simulink model "adaptive"  (R2018a)
settings: Solver=ode1  StartTime=0.0  StopTime=20  FixedStep=0.001  RelTol=1e-3
settings Model: Creator=mesih  LastModifiedBy=mesih

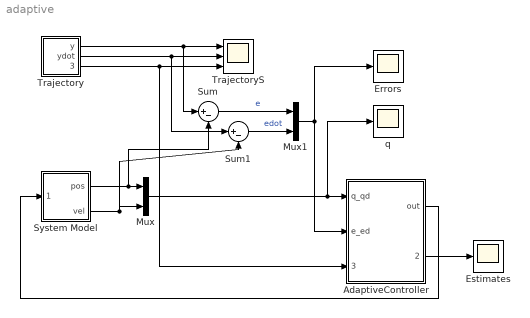
== system adaptive ==
  AdaptiveController : Subsystem
  Errors : Scope
  Estimates : Scope
  Mux : Mux  Inputs=2
  Mux1 : Mux  Inputs=2
  Sum : Sum  Inputs=|+-
  Sum1 : Sum  Inputs=|+-
  System Model : Subsystem
  Trajectory : Subsystem
  TrajectoryS : Scope  NumInputPorts=3
  q : Scope
  wires:
  Trajectory/1(y) -> Sum/1, TrajectoryS/1
  Trajectory/2(ydot) -> TrajectoryS/2, Sum1/1
  Trajectory/3(yddot) -> AdaptiveController/3(trajectory_dd), TrajectoryS/3
  System Model/1(pos) -> Sum/2, Mux/1
  System Model/2(vel) -> Mux/2, Sum1/2
  Sum/1 -> Mux1/1  "e"
  Sum1/1 -> Mux1/2  "edot"
  Mux1/1 -> AdaptiveController/2(e_ed), Errors/1
  AdaptiveController/1(out) -> System Model/1(input)
  Mux/1 -> q/1, AdaptiveController/1(q_qd)
  AdaptiveController/2("estimates ") -> Estimates/1

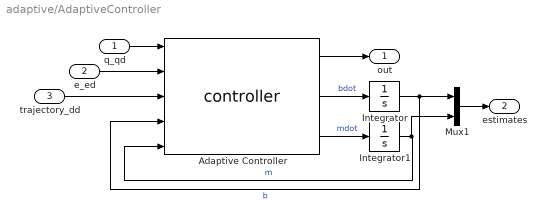
== system adaptive/AdaptiveController ==
  q_qd : Inport
  e_ed : Inport  Port=2
  trajectory_dd : Inport  Port=3
  Adaptive Controller : S-Function  FunctionName=controller  Parameters=1,10,5,3,0,0  SFunctionDeploymentMode=off  EnableBusSupport=off
  Integrator : Integrator
  Integrator1 : Integrator
  Mux1 : Mux  Inputs=2
  out : Outport
  "estimates " : Outport  Port=2
  wires:
  Adaptive Controller/1 -> out/1
  Integrator/1 -> Mux1/1, Adaptive Controller/4  "b"
  Integrator1/1 -> Mux1/2, Adaptive Controller/5  "m"
  Adaptive Controller/3 -> Integrator1/1  "mdot"
  q_qd/1 -> Adaptive Controller/1
  Adaptive Controller/2 -> Integrator/1  "bdot"
  trajectory_dd/1 -> Adaptive Controller/3
  e_ed/1 -> Adaptive Controller/2
  Mux1/1 -> "estimates "/1

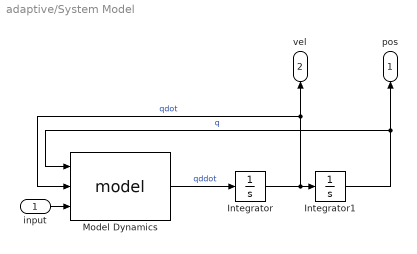
== system adaptive/System Model ==
  input : Inport
  Integrator : Integrator
  Integrator1 : Integrator
  Model Dynamics : S-Function  FunctionName=model  Parameters=2,1.5  SFunctionDeploymentMode=off  EnableBusSupport=off
  pos : Outport
  vel : Outport  Port=2
  wires:
  input/1 -> Model Dynamics/3
  Model Dynamics/1 -> Integrator/1  "qddot"
  Integrator1/1 -> pos/1, Model Dynamics/1  "q"
  Integrator/1 -> vel/1, Model Dynamics/2, Integrator1/1  "qdot"

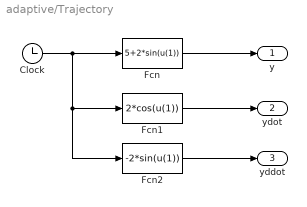
== system adaptive/Trajectory ==
  Clock : Clock
  Fcn : Fcn  Expr=5+2*sin(u(1))
  Fcn1 : Fcn  Expr=2*cos(u(1))
  Fcn2 : Fcn  Expr=-2*sin(u(1))
  y : Outport
  ydot : Outport  Port=2
  yddot : Outport  Port=3
  wires:
  Fcn1/1 -> ydot/1
  Fcn/1 -> y/1
  Clock/1 -> Fcn2/1, Fcn1/1, Fcn/1
  Fcn2/1 -> yddot/1
